simulink library "fmCopterDieterIndi_lib"  (R2018b)
settings: Solver=VariableStepAuto  StartTime=0.0  StopTime=10.0  RelTol=1e-3
undefined symbols (not defined in the file): cycle, DiscIntNeverNeededParam, fm_Traj, traj_empty
libraries: simulink x2, fmCopterAltHoldIndi_lib x2, cntrlPosNdi_lib x2, indi_lib x1, control_allocation_lib x1, ndi_lib x1, filters_lib x1, cntrlAttiRedIndi_lib x1, dspsigops x1, traj_lib x1
settings Model: Creator=Ybeyer  LastModifiedBy=eike
settings SFSimCC: SimUseLocalCustomCode=off
settings RTWCC: RTWUseLocalCustomCode=off
settings CodeAppCC: StateflowObjectComments=on

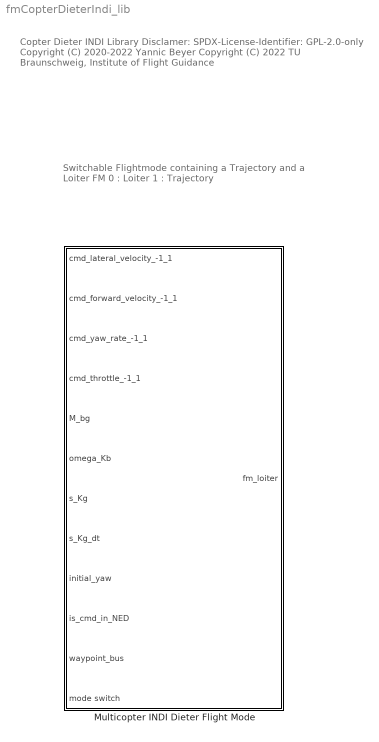
== system fmCopterDieterIndi_lib ==
  note: Switchable Flightmode
      | containing a Trajectory and a Loiter FM
      | 0 : Loiter
      | 1 : Trajectory
  note: Copter Dieter INDI Library
      |
      | Disclamer:
      | SPDX-License-Identifier: GPL-2.0-only
      |
      | Copyright (C) 2020-2022 Yannic Beyer
      | Copyright (C) 2022 TU Braunschweig, Institute of Flight Guidance
  Multicopter INDI Dieter Flight Mode : Subsystem  mask{fm=fm_Traj}
      mask prompts: fm "Multicopter INDI loiter flight  struct"
      mask DialogControl DescGroupVar Prompt: Multicopter INDI Loiter Flight Mode
      mask DialogControl DescTextVar Prompt: Loiter flight mode using the reduced attitude controller with INDI.
      mask DialogControl Control2 Prompt: To intialize the parameters struct see multicopterFlightModeLoiter.

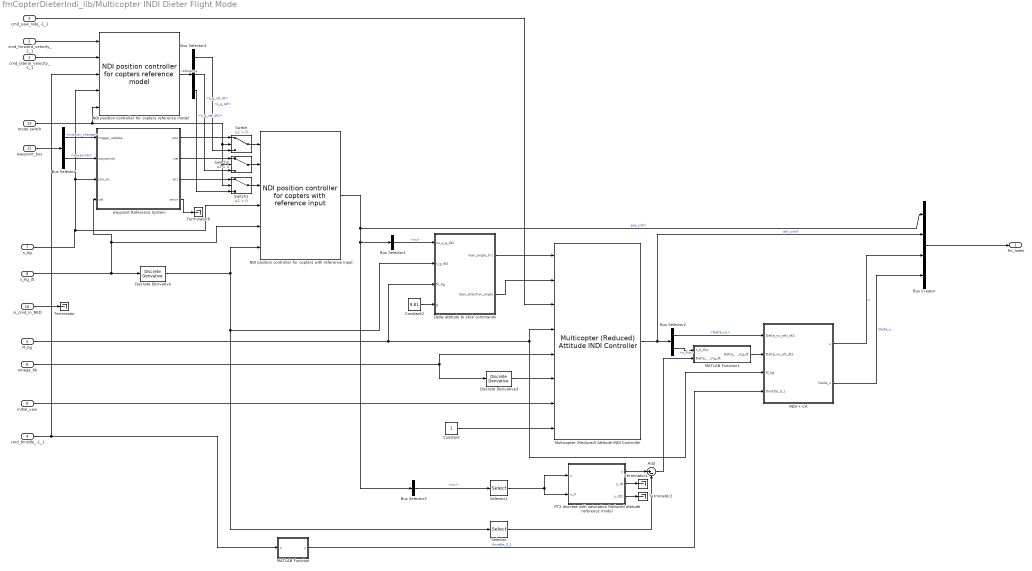
== system fmCopterDieterIndi_lib/Multicopter INDI Dieter Flight Mode ==
  cmd_lateral_velocity_-1_1 : Inport  SampleTime=fm.sample_time
  cmd_forward_velocity_-1_1 : Inport  Port=2  SampleTime=fm.sample_time
  cmd_yaw_rate_-1_1 : Inport  Port=3  SampleTime=fm.sample_time
  cmd_throttle_-1_1 : Inport  Port=4  SampleTime=fm.sample_time
  M_bg : Inport  Port=5  SampleTime=fm.sample_time
  omega_Kb : Inport  Port=6  SampleTime=fm.sample_time
  s_Kg : Inport  Port=7  SampleTime=fm.sample_time
  s_Kg_dt : Inport  Port=8  SampleTime=fm.sample_time
  initial_yaw : Inport  Port=9  SampleTime=fm.sample_time
  is_cmd_in_NED : Inport  Port=10  SampleTime=fm.sample_time
  waypoint_bus : Inport  Port=11
  mode switch : Inport  Port=12
  Add : Sum  Inputs=|+-
  Bus Creator : BusCreator  Inputs=4
  Bus Selector : BusSelector  OutputSignals=mission_change,waypoints
  Bus Selector1 : BusSelector  OutputSignals=pseudo_control.nu
  Bus Selector2 : BusSelector  OutputSignals=pseudo_control.Delta_ny,reference.reduced_attitude.n_flip
  Bus Selector3 : BusSelector  OutputSignals=pseudo_control.nu
  Bus Selector4 : BusSelector  OutputSignals=s_g_ref,s_g_ref_dt,s_g_ref_dt2
  Constant : Constant
  Constant2 : Constant  Value=9.81
  Delta attitude to stick commands : Subsystem
  Discrete Derivative : simulink/Discrete/Discrete Derivative  gainval=1.0  ICPrevScaledInput=0.0  OutMin=[]  OutMax=[]  OutDataType=fixdt(1, 16)  OutScaling=2^-10  DoSatur=off
  Discrete Derivative3 : simulink/Discrete/Discrete Derivative  gainval=1.0  ICPrevScaledInput=0.0  OutMin=[]  OutMax=[]  OutDataType=fixdt(1, 16)  OutScaling=2^-10  DoSatur=off
  INDI + CA : Subsystem
  MATLAB Function : MATLAB Function  TreatAsAtomicUnit=on
  MATLAB Function1 : MATLAB Function  TreatAsAtomicUnit=on
  Multicopter (Reduced) Attitude INDI Controller : cntrlAttiRedIndi_lib/Multicopter (Reduced) Attitude INDI Controller  atc=fm.atc  T=fm.motor_time_constant + 2./fm.sens_filt.omega
  NDI position controller for copters reference model : cntrlPosNdi_lib/NDI position controller for copters reference model  psc=fm.psc
      settings: SourceProductName=LADAC
  NDI position controller for copters with reference input : cntrlPosNdi_lib/NDI position controller for copters with reference input  psc=fm.psc  T_inner_loop=2./fm.atc.rm.leanfreq + fm.motor_time_constant + 2./fm.sens_filt.omega
      settings: SourceProductName=LADAC
  PT2 discrete with saturation Reduced attitude reference model : Subsystem  mask{omega=fm.atc.rm.leanfreq, d=fm.atc.rm.leandamp, x_dt2_max=inf, x_dt2_min=-inf, x_dt_max=inf, x_dt_min=-inf, x_max=inf, x_min=-inf, x_init=0, x_dt_init=0}
      mask prompts: omega "Natural frequency"; d "Damping ratio"; x_dt2_max "Maximum acceleration"; x_dt2_min "Minimum acceleration"; x_dt_max "Maximum rate"; x_dt_min "Minimum rate"; x_max "Maximum position"; x_min "Minimum position"; x_init "Initial position"; x_dt_init "Initial rate"
  Selector : Selector  InputPortWidth=3  IndexOptions=Index vector (dialog)  Indices=3  OutputSizes=1
  Selector1 : Selector  InputPortWidth=3  IndexOptions=Index vector (dialog)  Indices=3  OutputSizes=1
  Switch : Switch  Criteria=u2 > Threshold
  Switch1 : Switch  Criteria=u2 > Threshold
  Switch2 : Switch  Criteria=u2 > Threshold
  Terminator{,1..2,6} (4 alike) : Terminator
  waypoint Reference System : Subsystem
  fm_loiter : Outport  SampleTime=fm.sample_time
  wires:
  s_Kg_dt/1 -> waypoint Reference System/4("vel "), NDI position controller for copters with reference input/5, Discrete Derivative/1
  Discrete Derivative/1 -> NDI position controller for copters with reference input/6, Selector/1, Delta attitude to stick commands/2(s_g_dt2)
  cmd_yaw_rate_-1_1/1 -> Multicopter (Reduced) Attitude INDI Controller/3
  Constant/1 -> Multicopter (Reduced) Attitude INDI Controller/8
  s_Kg/1 -> waypoint Reference System/3(pos_ac), NDI position controller for copters reference model/4, NDI position controller for copters with reference input/4
  omega_Kb/1 -> Discrete Derivative3/1, Multicopter (Reduced) Attitude INDI Controller/5
  NDI position controller for copters with reference input/1 -> Bus Selector3/1, Bus Selector1/1, Bus Creator/1  "pos_cntrl"
  M_bg/1 -> Multicopter (Reduced) Attitude INDI Controller/4, INDI + CA/3(M_bg), Delta attitude to stick commands/3(M_bg)
  initial_yaw/1 -> Multicopter (Reduced) Attitude INDI Controller/7
  Bus Selector1/1 -> Delta attitude to stick commands/1(nu_s_g_dt2)  "<nu>"
  Bus Creator/1 -> fm_loiter/1
  is_cmd_in_NED/1 -> Terminator/1
  Multicopter (Reduced) Attitude INDI Controller/1 -> Bus Selector2/1, Bus Creator/2  "atti_cntrl"
  Bus Selector3/1 -> Selector1/1  "<nu>"
  Discrete Derivative3/1 -> Multicopter (Reduced) Attitude INDI Controller/6
  Delta attitude to stick commands/2(lean_direction_angle) -> Multicopter (Reduced) Attitude INDI Controller/2
  Delta attitude to stick commands/1(lean_angle_0-1) -> Multicopter (Reduced) Attitude INDI Controller/1
  MATLAB Function/1(y) -> INDI + CA/4(throttle_0_1)  "throttle_0_1"
  INDI + CA/1(u) -> Bus Creator/3  "u"
  INDI + CA/2(Delta_u) -> Bus Creator/4  "Delta_u"
  cmd_throttle_-1_1/1 -> NDI position controller for copters reference model/3, MATLAB Function/1(u)
  Bus Selector2/1 -> INDI + CA/1(Delta_nu_atti_dt2)  "<Delta_ny>"
  MATLAB Function1/1(Delta_nu_w_Kg_dt) -> INDI + CA/2(Delta_nu_alt_dt2)
  Bus Selector2/2 -> MATLAB Function1/1(n_b_flip)  "<n_flip>"
  Constant2/1 -> Delta attitude to stick commands/4(g)
  Selector/1 -> Add/2
  PT2 discrete with saturation Reduced attitude reference model/2(y_dt) -> Terminator1/1
  PT2 discrete with saturation Reduced attitude reference model/3(y_dt2) -> Terminator2/1
  Selector1/1 -> PT2 discrete with saturation Reduced attitude reference model/1(u), PT2 discrete with saturation Reduced attitude reference model/2(u_0)
  Add/1 -> MATLAB Function1/2("Delta_nu_w_Kg_dt ")
  PT2 discrete with saturation Reduced attitude reference model/1(y) -> Add/1
  waypoint Reference System/3(acc) -> Switch1/1
  waypoint Reference System/2(vel) -> Switch2/1
  waypoint Reference System/4(error) -> Terminator6/1
  cmd_forward_velocity_-1_1/1 -> NDI position controller for copters reference model/1
  cmd_lateral_velocity_-1_1/1 -> NDI position controller for copters reference model/2
  waypoint_bus/1 -> Bus Selector/1
  Bus Selector/1 -> waypoint Reference System/1(trigger_update)  "<mission_change>"
  Bus Selector/2 -> waypoint Reference System/2(waypoints)  "<waypoints>"
  NDI position controller for copters reference model/1 -> Bus Selector4/1  "reference"
  Switch/1 -> NDI position controller for copters with reference input/1
  Switch2/1 -> NDI position controller for copters with reference input/2
  Switch1/1 -> NDI position controller for copters with reference input/3
  Bus Selector4/1 -> Switch/3  "<s_g_ref>"
  Bus Selector4/2 -> Switch2/3  "<s_g_ref_dt>"
  Bus Selector4/3 -> Switch1/3  "<s_g_ref_dt2>"
  mode switch/1 -> NDI position controller for copters reference model/5, Switch1/2, Switch2/2, Switch/2
  waypoint Reference System/1(pos) -> Switch/1

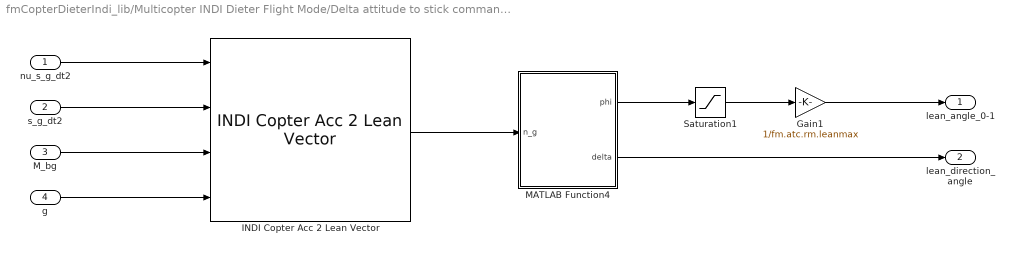
== system fmCopterDieterIndi_lib/Multicopter INDI Dieter Flight Mode/Delta attitude to stick commands ==
  nu_s_g_dt2 : Inport
  s_g_dt2 : Inport  Port=2
  M_bg : Inport  Port=3
  g : Inport  Port=4
  Gain1 : Gain  Gain=1/fm.atc.rm.leanmax
  INDI Copter Acc 2 Lean Vector : indi_lib/INDI Copter Acc 2 Lean Vector  SystemSampleTime=-1
      settings: SourceProductName=LADAC
  MATLAB Function4 : MATLAB Function  TreatAsAtomicUnit=on
  Saturation1 : Saturate  UpperLimit=fm.atc.rm.leanmax  LowerLimit=0
  lean_angle_0-1 : Outport
  lean_direction_angle : Outport  Port=2
  wires:
  M_bg/1 -> INDI Copter Acc 2 Lean Vector/3
  s_g_dt2/1 -> INDI Copter Acc 2 Lean Vector/2
  g/1 -> INDI Copter Acc 2 Lean Vector/4
  MATLAB Function4/1(phi) -> Saturation1/1
  Saturation1/1 -> Gain1/1
  nu_s_g_dt2/1 -> INDI Copter Acc 2 Lean Vector/1
  Gain1/1 -> lean_angle_0-1/1
  MATLAB Function4/2(delta) -> lean_direction_angle/1
  INDI Copter Acc 2 Lean Vector/1 -> MATLAB Function4/1(n_g)

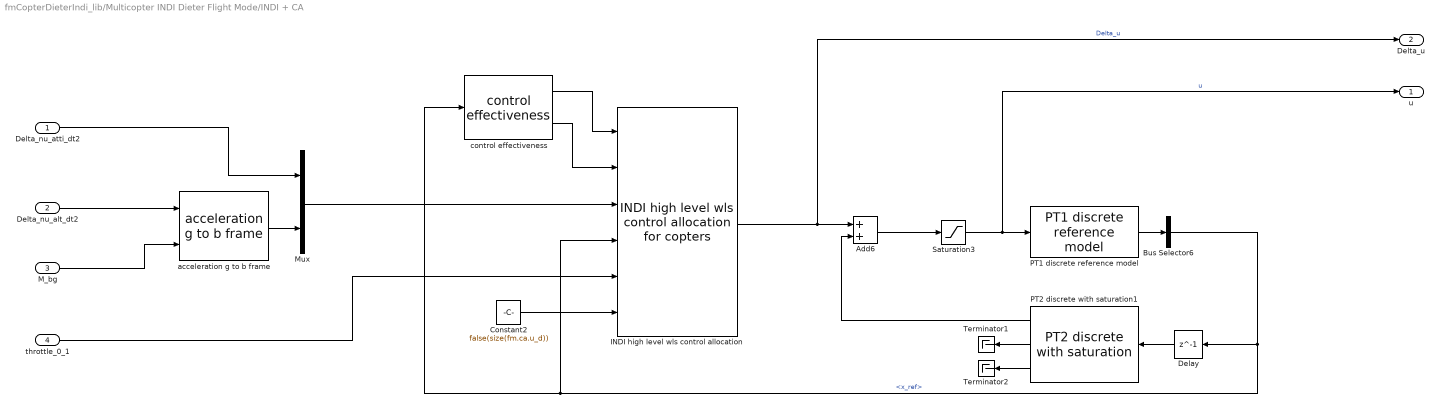
== system fmCopterDieterIndi_lib/Multicopter INDI Dieter Flight Mode/INDI + CA ==
  Delta_nu_atti_dt2 : Inport
  Delta_nu_alt_dt2 : Inport  Port=2
  M_bg : Inport  Port=3
  throttle_0_1 : Inport  Port=4
  Add6 : Sum
  Bus Selector6 : BusSelector  OutputSignals=x_ref
  Constant2 : Constant  Value=false(size(fm.ca.u_d))
  Delay : Delay  DelayLength=1
  INDI high level wls control allocation : control_allocation_lib/INDI high level wls control allocation for copters  ca=fm.ca  is_Delta_W_v_check=off  is_W_check=off  is_iter_check=off
  Mux : Mux  Inputs=2
  PT1 discrete reference model : ndi_lib/PT1 discrete reference model  T=fm.motor_time_constant  x_max=inf  x_min=-inf  x_dt_max=inf  x_dt_min=-inf  x_init=0
      settings: SourceProductName=LADAC
  PT2 discrete with saturation1 : filters_lib/PT2 discrete with saturation  omega=fm.sens_filt.omega  d=fm.sens_filt.D  x_dt2_max=inf  x_dt2_min=-inf  x_dt_max=inf  x_dt_min=-inf  x_max=inf  x_min=-inf  x_init=0  x_dt_init=0
      settings: SourceProductName=LADAC
  Saturation3 : Saturate  UpperLimit=fm.ca.u_max  LowerLimit=fm.ca.u_min
  Terminator1 : Terminator
  Terminator2 : Terminator
  acceleration g to b frame : fmCopterAltHoldIndi_lib/Multicopter Altitude Hold Flight Mode with INDI and reduced attitude control/acceleration g to b frame  SystemSampleTime=-1
      settings: SourceProductName=LADAC
  control effectiveness : fmCopterAltHoldIndi_lib/Multicopter Altitude Hold Flight Mode with INDI and reduced attitude control/control effectiveness  SystemSampleTime=-1
      settings: SourceProductName=LADAC
  u : Outport
  Delta_u : Outport  Port=2  PortDimensions=4
  wires:
  PT2 discrete with saturation1/1 -> Add6/2
  Mux/1 -> INDI high level wls control allocation/3
  Saturation3/1 -> u/1, PT1 discrete reference model/1  "u"
  INDI high level wls control allocation/1 -> Delta_u/1, Add6/1  "Delta_u"
  Delay/1 -> PT2 discrete with saturation1/1
  throttle_0_1/1 -> INDI high level wls control allocation/5
  Bus Selector6/1 -> Delay/1, control effectiveness/1, INDI high level wls control allocation/4  "<x_ref>"
  control effectiveness/1 -> INDI high level wls control allocation/1
  Constant2/1 -> INDI high level wls control allocation/6
  PT2 discrete with saturation1/2 -> Terminator1/1
  PT2 discrete with saturation1/3 -> Terminator2/1
  PT1 discrete reference model/1 -> Bus Selector6/1
  Add6/1 -> Saturation3/1
  Delta_nu_atti_dt2/1 -> Mux/1
  acceleration g to b frame/1 -> Mux/2
  Delta_nu_alt_dt2/1 -> acceleration g to b frame/1
  M_bg/1 -> acceleration g to b frame/2
  control effectiveness/2 -> INDI high level wls control allocation/2

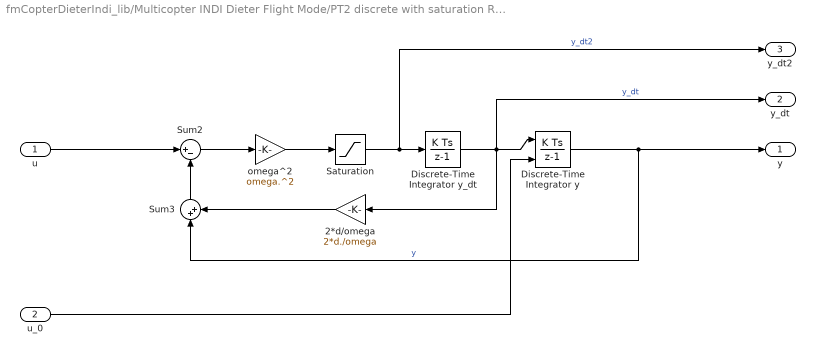
== system fmCopterDieterIndi_lib/Multicopter INDI Dieter Flight Mode/PT2 discrete with saturation Reduced attitude reference model ==
  u : Inport
  u_0 : Inport  Port=2
  2*d/omega : Gain  Gain=2*d./omega
  Discrete-Time Integrator y : DiscreteIntegrator  InitialConditionSource=external  InitialCondition=x_init  SampleTime=-1  OutDataTypeStr=Inherit: Inherit via back propagation  LimitOutput=on  UpperSaturationLimit=x_max  LowerSaturationLimit=x_min  ICPrevOutput=DiscIntNeverNeededParam  ICPrevScaledInput=DiscIntNeverNeededParam
  Discrete-Time Integrator y_dt : DiscreteIntegrator  InitialCondition=x_dt_init  SampleTime=-1  OutDataTypeStr=Inherit: Inherit via back propagation  LimitOutput=on  UpperSaturationLimit=x_dt_max  LowerSaturationLimit=x_dt_min  ICPrevOutput=DiscIntNeverNeededParam  ICPrevScaledInput=DiscIntNeverNeededParam
  Saturation : Saturate  UpperLimit=x_dt2_max  LowerLimit=x_dt2_min
  Sum2 : Sum  Inputs=|+-
  Sum3 : Sum  Inputs=|++
  omega^2 : Gain  Gain=omega.^2
  y : Outport
  y_dt : Outport  Port=2
  y_dt2 : Outport  Port=3
  wires:
  u_0/1 -> Discrete-Time Integrator y/2
  Discrete-Time Integrator y_dt/1 -> Discrete-Time Integrator y/1, y_dt/1, 2*d/omega/1  "y_dt"
  Discrete-Time Integrator y/1 -> y/1, Sum3/1  "y"
  Sum2/1 -> omega^2/1
  2*d/omega/1 -> Sum3/2
  u/1 -> Sum2/1
  Sum3/1 -> Sum2/2
  omega^2/1 -> Saturation/1
  Saturation/1 -> Discrete-Time Integrator y_dt/1, y_dt2/1  "y_dt2"

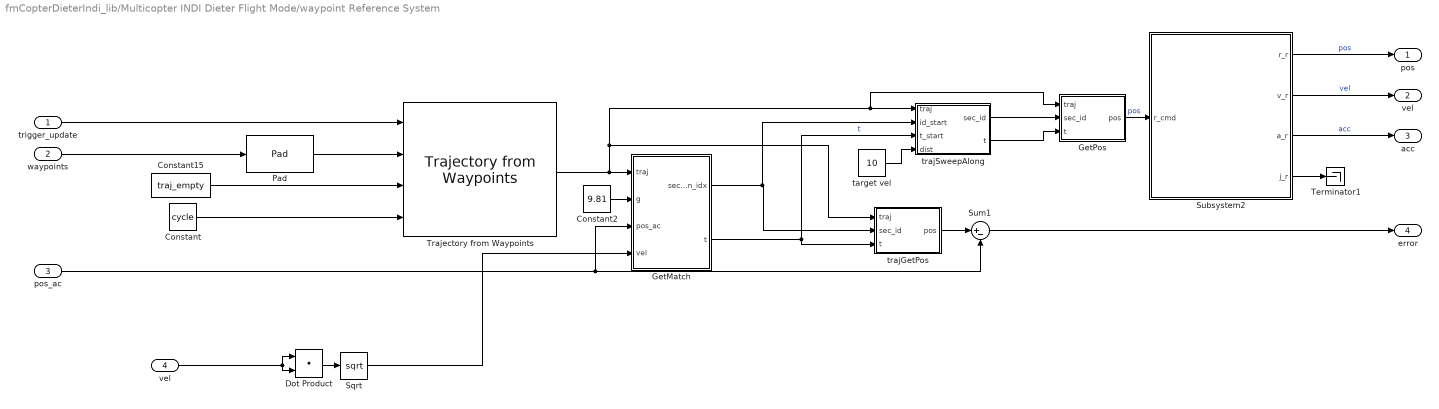
== system fmCopterDieterIndi_lib/Multicopter INDI Dieter Flight Mode/waypoint Reference System ==
  trigger_update : Inport
  waypoints : Inport  Port=2
  pos_ac : Inport  Port=3
  "vel " : Inport  Port=4
  Constant : Constant  Value=cycle
  Constant15 : Constant  Value=traj_empty  OutDataTypeStr=Bus: trajectoryBus
  Constant2 : Constant  Value=9.81  OutDataTypeStr=double
  Dot Product : DotProduct  InputSameDT=on  OutDataTypeStr=Inherit: Inherit via internal rule
  GetMatch : MATLAB Function  TreatAsAtomicUnit=on
  "GetPos " : MATLAB Function  TreatAsAtomicUnit=on
  Pad : dspsigops/Pad  padAlong=Columns and rows  dimsToPad=1  valSrc=Specify via dialog  padVal=0  spec=Output size  padNumOutRowsSpecMethod=User-specified  numOutRows=3  padNumOutColsSpecMethod=User-specified  numOutCols=6  isVarDimsMode=off  padBeginning=0  padEnd=0  outSizeMode=User-specified  outSize=1  padSigAt=End  trunc_flag=None  roundingMode=Floor  overflowMode=off  truncOrWrapMode=Truncate  wrap_flag=None
      settings: SourceProductName=DSP System Toolbox  SourceProductBaseCode=DS
  Sqrt : Sqrt  SaturateOnIntegerOverflow=on
  Subsystem2 : Subsystem
  Sum1 : Sum  Inputs=|+-
  Terminator1 : Terminator
  Trajectory from Waypoints : traj_lib/Trajectory from Waypoints
      settings: SourceProductName=LADAC
  target vel : Constant  Value=10
  trajGetPos : MATLAB Function  TreatAsAtomicUnit=on
  trajSweepAlong : MATLAB Function  TreatAsAtomicUnit=on
  pos : Outport
  vel : Outport  Port=2
  acc : Outport  Port=3
  error : Outport  Port=4
  wires:
  Sum1/1 -> error/1
  trajGetPos/1(pos) -> Sum1/1
  waypoints/1 -> Pad/1
  "GetPos "/1(pos) -> Subsystem2/1(r_cmd)  "pos"
  Sqrt/1 -> GetMatch/4(vel)
  pos_ac/1 -> GetMatch/3(pos_ac), Sum1/2
  trigger_update/1 -> Trajectory from Waypoints/1
  GetMatch/1(section_idx) -> trajSweepAlong/2(id_start), trajGetPos/2(sec_id)
  "vel "/1 -> Dot Product/2, Dot Product/1
  Subsystem2/3(a_r) -> acc/1  "acc"
  Subsystem2/2(v_r) -> vel/1  "vel"
  Subsystem2/1(r_r) -> pos/1  "pos"
  Constant/1 -> Trajectory from Waypoints/4
  Constant2/1 -> GetMatch/2(g)
  GetMatch/2(t) -> trajGetPos/3(t), trajSweepAlong/3(t_start)  "t"
  Dot Product/1 -> Sqrt/1
  trajSweepAlong/1(sec_id) -> "GetPos "/2(sec_id)
  target vel/1 -> trajSweepAlong/4(dist)
  Subsystem2/4(j_r) -> Terminator1/1
  trajSweepAlong/2(t) -> "GetPos "/3(t)
  Constant15/1 -> Trajectory from Waypoints/3
  Pad/1 -> Trajectory from Waypoints/2
  Trajectory from Waypoints/1 -> "GetPos "/1(traj), trajSweepAlong/1(traj), trajGetPos/1(traj), GetMatch/1(traj)

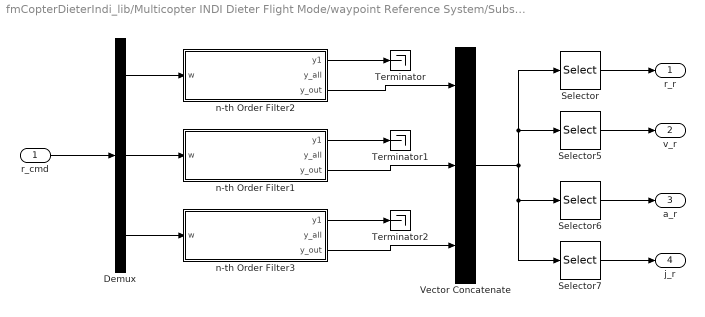
== system fmCopterDieterIndi_lib/Multicopter INDI Dieter Flight Mode/waypoint Reference System/Subsystem2 ==
  r_cmd : Inport
  Demux : Demux  Outputs=3
  Selector : Selector  InputPortWidth=12  IndexOptions=Index vector (dialog)  Indices=1:4:12  OutputSizes=1
  Selector5 : Selector  InputPortWidth=12  IndexOptions=Index vector (dialog)  Indices=2:4:12  OutputSizes=1
  Selector6 : Selector  InputPortWidth=12  IndexOptions=Index vector (dialog)  Indices=3:4:12  OutputSizes=1
  Selector7 : Selector  InputPortWidth=12  IndexOptions=Index vector (dialog)  Indices=4:4:12  OutputSizes=1
  Terminator : Terminator
  Terminator1 : Terminator
  Terminator2 : Terminator
  Vector Concatenate : Concatenate  NumInputs=3
  n-th Order Filter1 : Subsystem  mask{order=5, omega=6, output_order=4, use_inital_value=on}
      mask prompts: order "Filter order"; omega "Filter omega"; output_order "Outout Order"; use_inital_value "Start steady-state"
      mask init:
      | ss_model.order = order;
      | ss_model.omega = omega;
      | 
      | ss_model.K = ndiFeedbackGainPlace( -ss_model.omega*ones(ss_model.order,1), 0)
      | ss_model.A = diag(ones(ss_model.order-1,1),1)
      | ss_model.A(ss_model.order,:) = -ss_model.K';
      | 
      | ss_model.B = zeros(ss_model.order);
      | ss_model.C = eye(ss_model.order);
      | ss_model.D = zeros(ss_model.order);
      | 
      | ss_model.B(ss_model.order,ss_model.order) = ss_model.K(1);
  n-th Order Filter2 : Subsystem  mask{order=5, omega=6, output_order=4, use_inital_value=on}
      mask prompts: order "Filter order"; omega "Filter omega"; output_order "Outout Order"; use_inital_value "Start steady-state"
      mask init: same as fmCopterDieterIndi_lib/Multicopter INDI Dieter Flight Mode/waypoint Reference System/Subsystem2/n-th Order Filter1
  n-th Order Filter3 : Subsystem  mask{order=5, omega=6, output_order=4, use_inital_value=on}
      mask prompts: order "Filter order"; omega "Filter omega"; output_order "Outout Order"; use_inital_value "Start steady-state"
      mask init: same as fmCopterDieterIndi_lib/Multicopter INDI Dieter Flight Mode/waypoint Reference System/Subsystem2/n-th Order Filter1
  r_r : Outport
  v_r : Outport  Port=2
  a_r : Outport  Port=3
  j_r : Outport  Port=4
  wires:
  Selector7/1 -> j_r/1
  Selector5/1 -> v_r/1
  r_cmd/1 -> Demux/1
  Selector/1 -> r_r/1
  Demux/1 -> n-th Order Filter2/1(w)
  n-th Order Filter3/1(y1) -> Terminator2/1
  n-th Order Filter2/1(y1) -> Terminator/1
  Selector6/1 -> a_r/1
  Demux/3 -> n-th Order Filter3/1(w)
  Demux/2 -> n-th Order Filter1/1(w)
  n-th Order Filter1/1(y1) -> Terminator1/1
  Vector Concatenate/1 -> Selector5/1, Selector/1, Selector7/1, Selector6/1
  n-th Order Filter2/3(y_out) -> Vector Concatenate/1
  n-th Order Filter3/3(y_out) -> Vector Concatenate/3
  n-th Order Filter1/3(y_out) -> Vector Concatenate/2

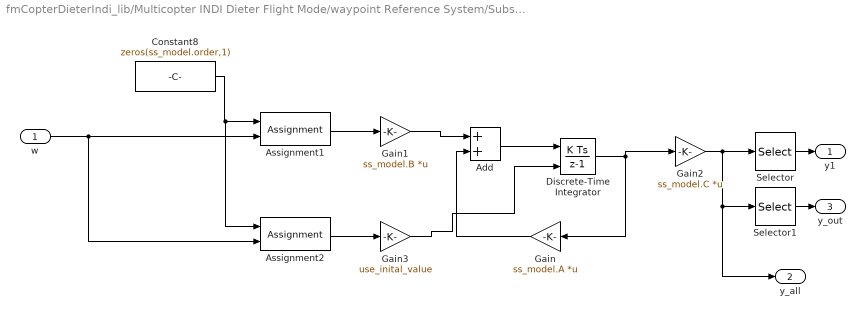
== system fmCopterDieterIndi_lib/Multicopter INDI Dieter Flight Mode/waypoint Reference System/Subsystem2/n-th Order Filter1 ==
  w : Inport
  Add : Sum
  Assignment1 : Assignment  DiagnosticForDimensions=Warning  IndexOptions=Index vector (dialog)  Indices=ss_model.order  OutputSizes=1
  Assignment2 : Assignment  DiagnosticForDimensions=Warning  IndexOptions=Index vector (dialog)  Indices=1  OutputSizes=1
  Constant8 : Constant  Value=zeros(ss_model.order,1)  VectorParams1D=off
  Discrete-Time Integrator : DiscreteIntegrator  InitialConditionSource=external  SampleTime=-1  ICPrevOutput=DiscIntNeverNeededParam  ICPrevScaledInput=DiscIntNeverNeededParam
  Gain : Gain  Gain=ss_model.A  Multiplication=Matrix(K*u)
  Gain1 : Gain  Gain=ss_model.B  Multiplication=Matrix(K*u)
  Gain2 : Gain  Gain=ss_model.C  Multiplication=Matrix(K*u)
  Gain3 : Gain  Gain=use_inital_value
  Selector : Selector  InputPortWidth=ss_model.order  IndexOptions=Index vector (dialog)  Indices=1  OutputSizes=1
  Selector1 : Selector  InputPortWidth=ss_model.order  IndexOptions=Index vector (dialog)  Indices=1:output_order  OutputSizes=1
  y1 : Outport
  y_all : Outport  Port=2
  y_out : Outport  Port=3
  wires:
  Constant8/1 -> Assignment2/1, Assignment1/1
  w/1 -> Assignment2/2, Assignment1/2
  Selector/1 -> y1/1
  Discrete-Time Integrator/1 -> Gain2/1, Gain/1
  Gain1/1 -> Add/1
  Assignment1/1 -> Gain1/1
  Add/1 -> Discrete-Time Integrator/1
  Gain2/1 -> Selector1/1, y_all/1, Selector/1
  Gain/1 -> Add/2
  Assignment2/1 -> Gain3/1
  Gain3/1 -> Discrete-Time Integrator/2
  Selector1/1 -> y_out/1

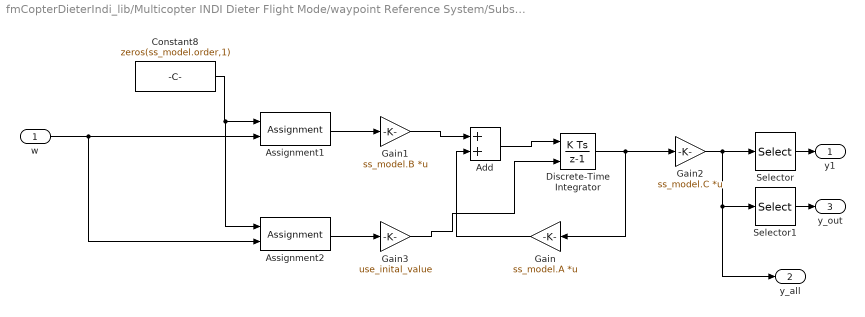
== system fmCopterDieterIndi_lib/Multicopter INDI Dieter Flight Mode/waypoint Reference System/Subsystem2/n-th Order Filter2 ==
  w : Inport
  Add : Sum
  Assignment1 : Assignment  DiagnosticForDimensions=Warning  IndexOptions=Index vector (dialog)  Indices=ss_model.order  OutputSizes=1
  Assignment2 : Assignment  DiagnosticForDimensions=Warning  IndexOptions=Index vector (dialog)  Indices=1  OutputSizes=1
  Constant8 : Constant  Value=zeros(ss_model.order,1)  VectorParams1D=off
  Discrete-Time Integrator : DiscreteIntegrator  InitialConditionSource=external  SampleTime=-1  ICPrevOutput=DiscIntNeverNeededParam  ICPrevScaledInput=DiscIntNeverNeededParam
  Gain : Gain  Gain=ss_model.A  Multiplication=Matrix(K*u)
  Gain1 : Gain  Gain=ss_model.B  Multiplication=Matrix(K*u)
  Gain2 : Gain  Gain=ss_model.C  Multiplication=Matrix(K*u)
  Gain3 : Gain  Gain=use_inital_value
  Selector : Selector  InputPortWidth=ss_model.order  IndexOptions=Index vector (dialog)  Indices=1  OutputSizes=1
  Selector1 : Selector  InputPortWidth=ss_model.order  IndexOptions=Index vector (dialog)  Indices=1:output_order  OutputSizes=1
  y1 : Outport
  y_all : Outport  Port=2
  y_out : Outport  Port=3
  wires:
  Constant8/1 -> Assignment2/1, Assignment1/1
  w/1 -> Assignment2/2, Assignment1/2
  Selector/1 -> y1/1
  Discrete-Time Integrator/1 -> Gain2/1, Gain/1
  Gain1/1 -> Add/1
  Assignment1/1 -> Gain1/1
  Add/1 -> Discrete-Time Integrator/1
  Gain2/1 -> Selector1/1, y_all/1, Selector/1
  Gain/1 -> Add/2
  Assignment2/1 -> Gain3/1
  Gain3/1 -> Discrete-Time Integrator/2
  Selector1/1 -> y_out/1

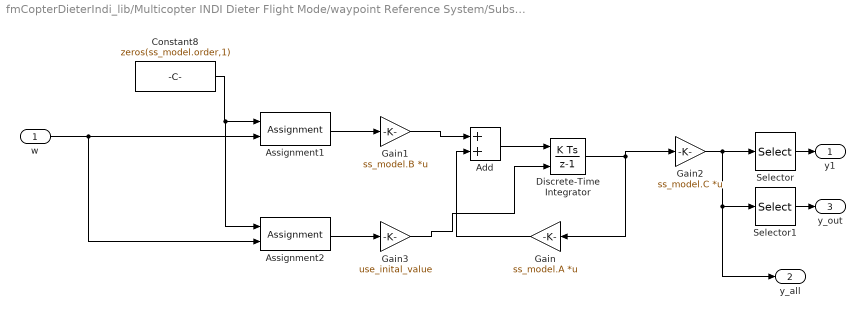
== system fmCopterDieterIndi_lib/Multicopter INDI Dieter Flight Mode/waypoint Reference System/Subsystem2/n-th Order Filter3 ==
  w : Inport
  Add : Sum
  Assignment1 : Assignment  DiagnosticForDimensions=Warning  IndexOptions=Index vector (dialog)  Indices=ss_model.order  OutputSizes=1
  Assignment2 : Assignment  DiagnosticForDimensions=Warning  IndexOptions=Index vector (dialog)  Indices=1  OutputSizes=1
  Constant8 : Constant  Value=zeros(ss_model.order,1)  VectorParams1D=off
  Discrete-Time Integrator : DiscreteIntegrator  InitialConditionSource=external  SampleTime=-1  ICPrevOutput=DiscIntNeverNeededParam  ICPrevScaledInput=DiscIntNeverNeededParam
  Gain : Gain  Gain=ss_model.A  Multiplication=Matrix(K*u)
  Gain1 : Gain  Gain=ss_model.B  Multiplication=Matrix(K*u)
  Gain2 : Gain  Gain=ss_model.C  Multiplication=Matrix(K*u)
  Gain3 : Gain  Gain=use_inital_value
  Selector : Selector  InputPortWidth=ss_model.order  IndexOptions=Index vector (dialog)  Indices=1  OutputSizes=1
  Selector1 : Selector  InputPortWidth=ss_model.order  IndexOptions=Index vector (dialog)  Indices=1:output_order  OutputSizes=1
  y1 : Outport
  y_all : Outport  Port=2
  y_out : Outport  Port=3
  wires:
  Constant8/1 -> Assignment2/1, Assignment1/1
  w/1 -> Assignment2/2, Assignment1/2
  Selector/1 -> y1/1
  Discrete-Time Integrator/1 -> Gain2/1, Gain/1
  Gain1/1 -> Add/1
  Assignment1/1 -> Gain1/1
  Add/1 -> Discrete-Time Integrator/1
  Gain2/1 -> Selector1/1, y_all/1, Selector/1
  Gain/1 -> Add/2
  Assignment2/1 -> Gain3/1
  Gain3/1 -> Discrete-Time Integrator/2
  Selector1/1 -> y_out/1

== matlab function fmCopterDieterIndi_lib/Multicopter INDI Dieter Flight Mode/waypoint Reference System/trajGetPos ==
  data: traj input; pos output size=3; sec_id input; t input
function pos = trajGetPos(traj, sec_id,t)
sec = trajGetSection(traj,sec_id);
pos = trajSectionGetPos(sec,t);

== matlab function fmCopterDieterIndi_lib/Multicopter INDI Dieter Flight Mode/MATLAB Function1 ==
  data: n_b_flip input; Delta_nu_w_Kg_dt input; Delta_nu_w_Kg_dt output
function Delta_nu_w_Kg_dt = fcn( n_b_flip, Delta_nu_w_Kg_dt )

if n_b_flip(3) >= 0
    Delta_nu_w_Kg_dt(:) = 0;
end

end

== matlab function fmCopterDieterIndi_lib/Multicopter INDI Dieter Flight Mode/Delta attitude to stick commands/MATLAB Function4 ==
  data: n_g input; phi output; delta output
function [phi,delta] = leanVector2LeanAngles(n_g)
[phi,delta] = leanVector2LeanAngles(n_g);
end

== matlab function fmCopterDieterIndi_lib/Multicopter INDI Dieter Flight Mode/MATLAB Function ==
  data: u input; y output
function y = fcn(u)
y = 0.5*u+0.5;

== matlab function fmCopterDieterIndi_lib/Multicopter INDI Dieter Flight Mode/waypoint Reference System/trajSweepAlong ==
  data: traj input; sec_id output size=1; id_start input size=1; t_start input; dist input; t output size=1
function [sec_id,t] = trajSweepAlong(traj,id_start,t_start,dist)
[sec_id, t] = trajSweepAlong(traj,id_start,t_start,dist);

== matlab function fmCopterDieterIndi_lib/Multicopter INDI Dieter Flight Mode/waypoint Reference System/GetPos  ==
  data: traj input; pos output size=3; sec_id input; t input
function pos = trajGetPos(traj, sec_id,t)
sec = trajGetSection(traj,sec_id);
pos = trajSectionGetPos(sec,t);

== matlab function fmCopterDieterIndi_lib/Multicopter INDI Dieter Flight Mode/waypoint Reference System/GetMatch ==
  data: traj input size=1; section_idx output size=1; g input size=1; pos_ac input size=3; vel input size=1; t output size=1
function [section_idx, t]  = GetMatch(traj, g, pos_ac, vel)

[section_idx, ~, t] = trajGetMatch(traj,pos_ac,vel);
end
